simulink model "gear_verification_system"  (R2024a)
settings: Solver=VariableStepAuto  StartTime=0.0  StopTime=10.0  RelTol=1e-3
libraries: simulink x5
settings Model: Creator=admin  LastModifiedBy=admin

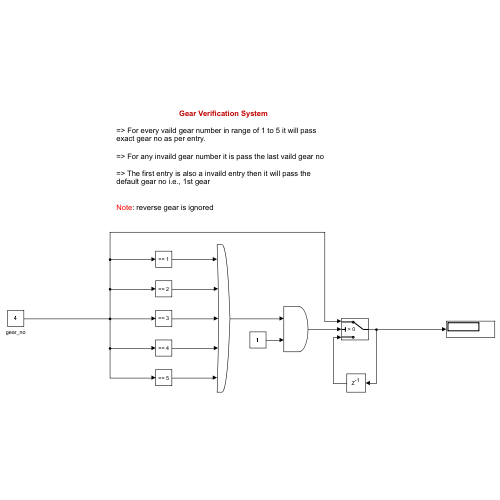
[thumbnail: Simulink's stored preview of the top-level diagram]
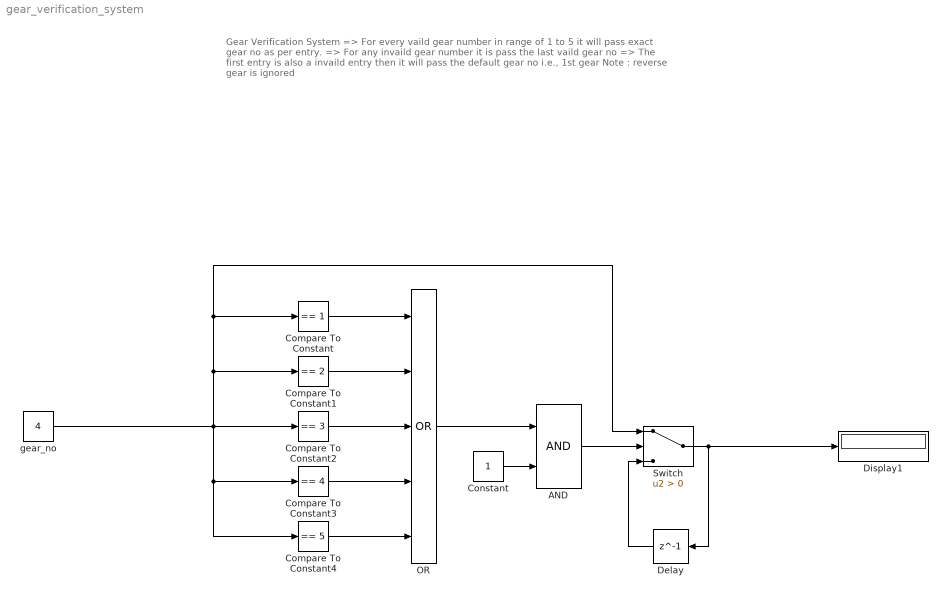
== system gear_verification_system ==
  note: Gear Verification System
      |
      | => For every vaild gear number in range of 1 to 5 it will pass exact gear no as per entry.
      |
      | => For any invaild gear number it is pass the last vaild gear no
      |
      | => The first entry is also a invaild entry then it will pass the default gear no i.e., 1st gear
      |
      | Note : reverse gear is ignored
  AND : Logic  IconShape=distinctive  AllPortsSameDT=off  OutDataTypeStr=boolean
  Compare To Constant : simulink/Logic and Bit Operations/Compare To Constant  relop===  const=1  OutDataTypeStr=boolean
  Compare To Constant1 : simulink/Logic and Bit Operations/Compare To Constant  relop===  const=2  OutDataTypeStr=boolean
  Compare To Constant2 : simulink/Logic and Bit Operations/Compare To Constant  relop===  const=3  OutDataTypeStr=boolean
  Compare To Constant3 : simulink/Logic and Bit Operations/Compare To Constant  relop===  const=4  OutDataTypeStr=boolean
  Compare To Constant4 : simulink/Logic and Bit Operations/Compare To Constant  relop===  const=5  OutDataTypeStr=boolean
  Constant : Constant
  Delay : Delay  DelayLength=1  InitialCondition=1
  Display1 : Display
  OR : Logic  Operator=OR  Inputs=5  IconShape=distinctive  AllPortsSameDT=off  OutDataTypeStr=boolean
  Switch : Switch  Criteria=u2 > Threshold  SaturateOnIntegerOverflow=off  InputSameDT=off
  gear_no : Constant  Value=4
  wires:
  Switch/1 -> Display1/1, Delay/1
  Delay/1 -> Switch/3
  Compare To Constant3/1 -> OR/4
  AND/1 -> Switch/2
  OR/1 -> AND/1
  Compare To Constant1/1 -> OR/2
  Constant/1 -> AND/2
  Compare To Constant/1 -> OR/1
  gear_no/1 -> Compare To Constant3/1, Compare To Constant4/1, Compare To Constant2/1, Compare To Constant1/1, Switch/1, Compare To Constant/1
  Compare To Constant4/1 -> OR/5
  Compare To Constant2/1 -> OR/3
